simulink model "ex_longlat_dynamics_with_tire"  (R2026a)
settings: Solver=VariableStepAuto
libraries: aerolibconvert2 x2
settings Model: Creator=doyeop  LastModifiedBy=doyeop

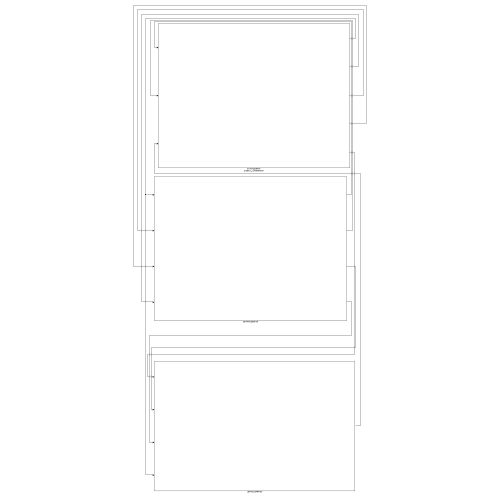
[thumbnail: Simulink's stored preview of the top-level diagram]
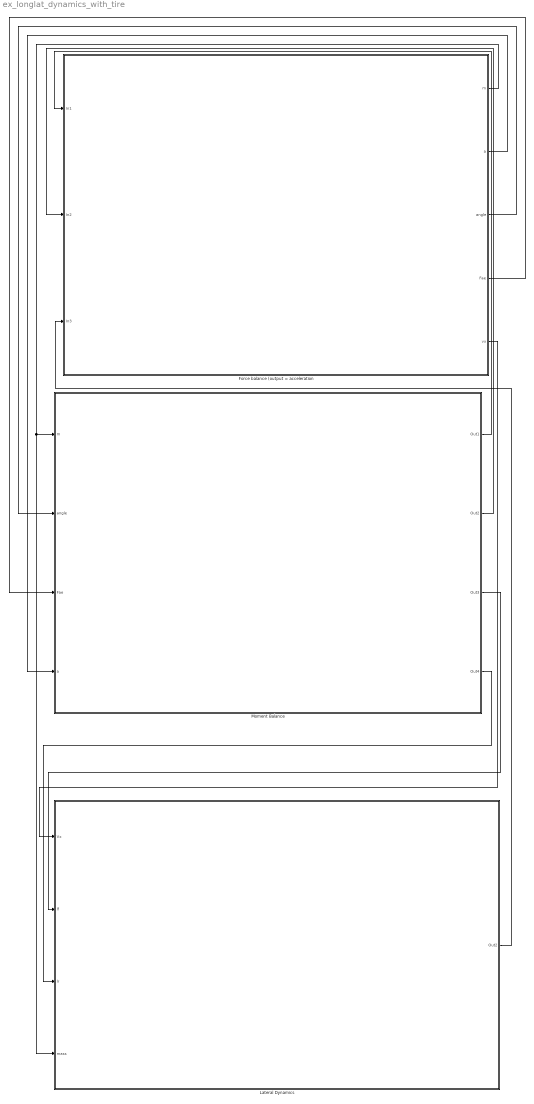
== system ex_longlat_dynamics_with_tire ==
  Force balance (output = acceleration : Subsystem
  Lateral Dynamics : Subsystem
  Moment Balance : Subsystem
  wires:
  Force balance (output = acceleration/1(m) -> Lateral Dynamics/4(mass), Moment Balance/1(m)
  Force balance (output = acceleration/2(a) -> Moment Balance/4(a)
  Force balance (output = acceleration/3(angle) -> Moment Balance/2(angle)
  Force balance (output = acceleration/4(Fae) -> Moment Balance/3(Fae)
  Moment Balance/1(Out1) -> Force balance (output = acceleration/1(In1)
  Moment Balance/2(Out2) -> Force balance (output = acceleration/2(In2)
  Force balance (output = acceleration/5(vx) -> Lateral Dynamics/1(Vx)
  Moment Balance/3(Out3) -> Lateral Dynamics/2(lf)
  Moment Balance/4(Out4) -> Lateral Dynamics/3(lr)
  Lateral Dynamics/1(Out2) -> Force balance (output = acceleration/3(In3)

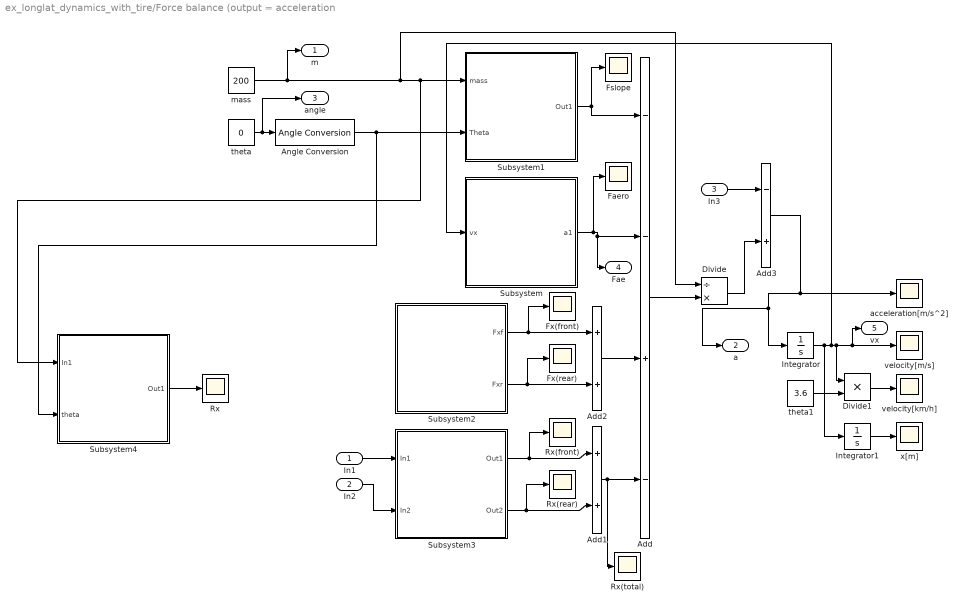
== system ex_longlat_dynamics_with_tire/Force balance (output = acceleration ==
  In1 : Inport
  In2 : Inport  Port=2
  In3 : Inport  Port=3
  Add : Sum  Inputs=--+-
  Add1 : Sum
  Add2 : Sum
  Add3 : Sum  Inputs=-+
  Angle Conversion : aerolibconvert2/Angle Conversion  IU=deg  OU=rad
  Divide : Product  Inputs=/*
  Divide1 : Product  Inputs=**
  Faero : Scope
      settings: ActiveDisplayYMinimum=-21.806973838724872  ActiveDisplayYMaximum=245.93181269445461  DataLoggingVariableName=ScopeData4
  Fslope : Scope
      settings: ActiveDisplayYMinimum=467.68768501992645  ActiveDisplayYMaximum=4126.826484026702  DataLoggingVariableName=ScopeData3
  Fx(front) : Scope
      settings: ActiveDisplayYMinimum=-0.77322383064043154  ActiveDisplayYMaximum=0.91988628090500946  DataLoggingVariableName=ScopeData5
  Fx(rear) : Scope
      settings: ActiveDisplayYMinimum=-0.77322383064043154  ActiveDisplayYMaximum=0.91988628090500946  DataLoggingVariableName=ScopeData10
  Integrator : Integrator
  Integrator1 : Integrator
  Rx : Scope
      settings: ActiveDisplayYMinimum=21.392000000000003  ActiveDisplayYMaximum=41.392  DataLoggingVariableName=ScopeData6
  Rx(front) : Scope
      settings: ActiveDisplayYMinimum=-1  ActiveDisplayYMaximum=1  DataLoggingVariableName=ScopeData11
  Rx(rear) : Scope
      settings: ActiveDisplayYMinimum=-1  ActiveDisplayYMaximum=1  DataLoggingVariableName=ScopeData12
  Rx(total) : Scope
      settings: ActiveDisplayYMinimum=26.459225679325527  ActiveDisplayYMaximum=38.083177364358953  DataLoggingVariableName=ScopeData13
  Subsystem : Subsystem
  Subsystem1 : Subsystem
  Subsystem2 : Subsystem
  Subsystem3 : Subsystem
  Subsystem4 : Subsystem
  acceleration[m/s^2] : Scope
      settings: ActiveDisplayYMinimum=-1  ActiveDisplayYMaximum=1
  mass : Constant  Value=200  SampleTime=-1
  theta : Constant  Value=0  SampleTime=-1
  theta1 : Constant  Value=3.6  SampleTime=-1
  velocity[km/h] : Scope
      settings: ActiveDisplayYMinimum=-12.890564976943338  ActiveDisplayYMaximum=101.85529757372632  DataLoggingVariableName=ScopeData7
  velocity[m/s] : Scope
      settings: ActiveDisplayYMinimum=-1  ActiveDisplayYMaximum=1
  x[m] : Scope
      settings: ActiveDisplayYMinimum=-1  ActiveDisplayYMaximum=1  DataLoggingVariableName=ScopeData2
  m : Outport
  a : Outport  Port=2
  angle : Outport  Port=3
  Fae : Outport  Port=4
  vx : Outport  Port=5
  wires:
  Divide1/1 -> velocity[km/h]/1
  Subsystem/1(a1) -> Faero/1, Add/2, Fae/1
  Integrator1/1 -> x[m]/1
  Add/1 -> Divide/2
  Angle Conversion/1 -> Subsystem4/2(theta), Subsystem1/2(Theta)
  mass/1 -> m/1, Divide/1, Subsystem4/1(In1), Subsystem1/1(mass)
  Subsystem2/1(Fxf) -> Add2/1, Fx(front)/1
  theta1/1 -> Divide1/2
  Integrator/1 -> Integrator1/1, Subsystem/1(vx), Divide1/1, vx/1, velocity[m/s]/1
  Subsystem1/1(Out1) -> Fslope/1, Add/1
  Subsystem4/1(Out1) -> Rx/1
  theta/1 -> angle/1, Angle Conversion/1
  Subsystem2/2(Fxr) -> Fx(rear)/1, Add2/2
  In1/1 -> Subsystem3/1(In1)
  In2/1 -> Subsystem3/2(In2)
  Add1/1 -> Add/4, Rx(total)/1
  Subsystem3/2(Out2) -> Rx(rear)/1, Add1/2
  Subsystem3/1(Out1) -> Rx(front)/1, Add1/1
  Add2/1 -> Add/3
  In3/1 -> Add3/1
  Divide/1 -> Add3/2
  Add3/1 -> acceleration[m/s^2]/1, a/1, Integrator/1

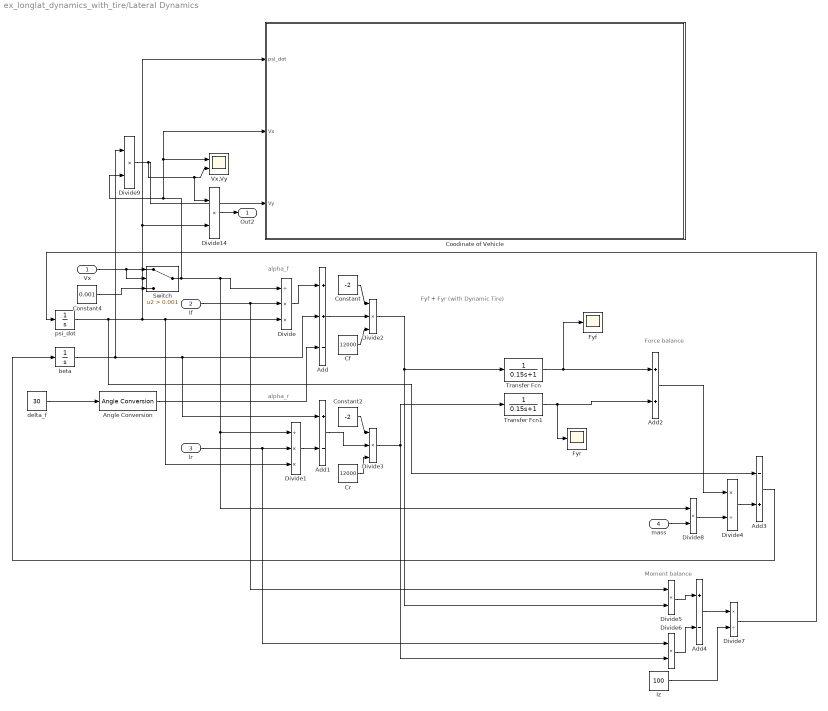
== system ex_longlat_dynamics_with_tire/Lateral Dynamics ==
  note: Moment balance
  note: Force balance
  note: Fyf + Fyr (with Dynamic Tire)
  note: alpha_r
  note: alpha_f
  Vx : Inport
  lf : Inport  Port=2
  lr : Inport  Port=3
  mass : Inport  Port=4
  Add : Sum  Inputs=++-
  Add1 : Sum  Inputs=+-
  Add2 : Sum
  Add3 : Sum  Inputs=-+
  Add4 : Sum  Inputs=+-
  Angle Conversion : aerolibconvert2/Angle Conversion  IU=deg  OU=rad
  Cf : Constant  Value=12000  SampleTime=-1
  Constant : Constant  Value=-2  SampleTime=-1
  Constant2 : Constant  Value=-2  SampleTime=-1
  Constant4 : Constant  Value=0.001
  Coodinate of Vehicle : Subsystem
  Cr : Constant  Value=12000  SampleTime=-1
  Divide : Product  Inputs=/**
  Divide1 : Product  Inputs=/**
  Divide{5..6,8..9,14} (5 alike) : Product  Inputs=**
  Divide2 : Product  Inputs=***
  Divide3 : Product  Inputs=***
  Divide4 : Product  Inputs=*/
  Divide7 : Product  Inputs=*/
  Fyf : Scope
      settings: ActiveDisplayYMinimum=-1407.4048741262529  ActiveDisplayYMaximum=11639.532558539519  DataLoggingVariableName=ScopeData14
  Fyr : Scope
      settings: ActiveDisplayYMinimum=-970.12534509010345  ActiveDisplayYMaximum=7745.6964021526865  DataLoggingVariableName=ScopeData15
  Iz : Constant  Value=100  SampleTime=-1
  Switch : Switch  Criteria=u2 > Threshold  Threshold=0.001  SaturateOnIntegerOverflow=off  InputSameDT=off
  Transfer Fcn : TransferFcn  Denominator=[0.15 1]
  Transfer Fcn1 : TransferFcn  Denominator=[0.15 1]
  Vx,Vy : Scope  NumInputPorts=2
      settings: ActiveDisplayYMinimum=-0.62237224027035509  ActiveDisplayYMaximum=5.6013501624331967  DataLoggingVariableName=ScopeData16
  beta : Integrator
  delta_f : Constant  Value=30
  psi_dot : Integrator
  Out2 : Outport
  wires:
  beta/1 -> Add/2, Add1/1, Divide9/1
  Divide/1 -> Add/1
  Angle Conversion/1 -> Add/3
  lr/1 -> Divide6/1, Divide1/2
  Divide1/1 -> Add1/2
  Constant/1 -> Divide2/1
  Add/1 -> Divide2/2
  Cf/1 -> Divide2/3
  Add1/1 -> Divide3/2
  Constant2/1 -> Divide3/1
  Cr/1 -> Divide3/3
  Divide2/1 -> Transfer Fcn/1, Divide5/2
  Divide3/1 -> Divide6/2, Transfer Fcn1/1
  Divide4/1 -> Add3/2
  Add3/1 -> beta/1
  lf/1 -> Divide5/1, Divide/2
  Divide5/1 -> Add4/1
  Divide6/1 -> Add4/2
  Add4/1 -> Divide7/1
  Iz/1 -> Divide7/2
  Divide7/1 -> psi_dot/1
  Vx/1 -> Switch/2, Switch/1
  Constant4/1 -> Switch/3
  mass/1 -> Divide8/2
  Divide8/1 -> Divide4/2
  Add2/1 -> Divide4/1
  delta_f/1 -> Angle Conversion/1
  Transfer Fcn/1 -> Fyf/1, Add2/1
  Transfer Fcn1/1 -> Fyr/1, Add2/2
  Switch/1 -> Divide8/1, Divide1/1, Divide/1, Divide9/2, Coodinate of Vehicle/2(Vx), Vx,Vy/1
  Divide9/1 -> Divide14/1, Vx,Vy/2, Coodinate of Vehicle/3(Vy)
  psi_dot/1 -> Add3/1, Divide14/2, Coodinate of Vehicle/1(psi_dot), Divide1/3, Divide/3
  Divide14/1 -> Out2/1

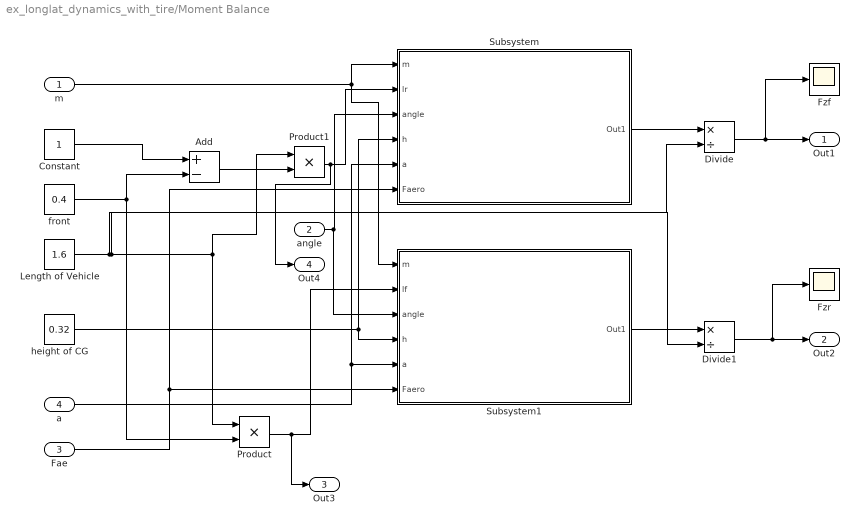
== system ex_longlat_dynamics_with_tire/Moment Balance ==
  m : Inport
  angle : Inport  Port=2
  Fae : Inport  Port=3
  a : Inport  Port=4
  Add : Sum  Inputs=+-
  Constant : Constant
  Divide : Product  Inputs=*/
  Divide1 : Product  Inputs=*/
  Fzf : Scope
      settings: ActiveDisplayYMinimum=684.79999999999961  ActiveDisplayYMaximum=684.80000000000007  DataLoggingVariableName=ScopeData8
  Fzr : Scope
      settings: DataLoggingVariableName=ScopeData9
  Length of Vehicle : Constant  Value=1.6  SampleTime=-1
  Product : Product
  Product1 : Product
  Subsystem : Subsystem
  Subsystem1 : Subsystem
  front : Constant  Value=0.4  SampleTime=-1
  height of CG : Constant  Value=0.32
  Out1 : Outport
  Out2 : Outport  Port=2
  Out3 : Outport  Port=3
  Out4 : Outport  Port=4
  wires:
  m/1 -> Subsystem1/1(m), Subsystem/1(m)
  angle/1 -> Subsystem1/3(angle), Subsystem/3(angle)
  front/1 -> Product/2, Add/2
  Constant/1 -> Add/1
  Length of Vehicle/1 -> Divide/2, Divide1/2, Product1/1, Product/1
  Add/1 -> Product1/2
  Product1/1 -> Out4/1, Subsystem/2(lr)
  height of CG/1 -> Subsystem/4(h), Subsystem1/4(h)
  a/1 -> Subsystem1/5(a), Subsystem/5(a)
  Fae/1 -> Subsystem1/6(Faero), Subsystem/6(Faero)
  Subsystem/1(Out1) -> Divide/1
  Subsystem1/1(Out1) -> Divide1/1
  Product/1 -> Out3/1, Subsystem1/2(lf)
  Divide/1 -> Out1/1, Fzf/1
  Divide1/1 -> Fzr/1, Out2/1

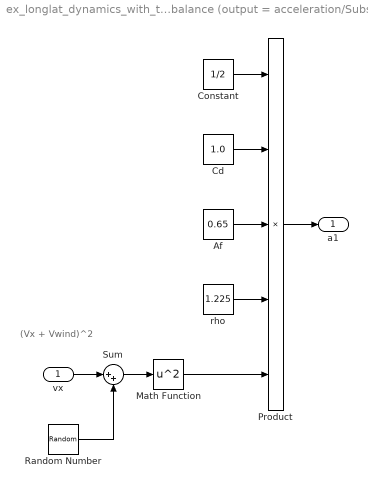
== system ex_longlat_dynamics_with_tire/Force balance (output = acceleration/Subsystem ==
  note: (Vx + Vwind)^2
  vx : Inport
  Af : Constant  Value=0.65  SampleTime=-1
  Cd : Constant  Value=1.0  SampleTime=-1
  Constant : Constant  Value=1/2  SampleTime=-1
  Math Function : Math  Operator=square
  Product : Product  Inputs=5
  Random Number : RandomNumber  Mean=3  Variance=0.5^2  SampleTime=0.1
  Sum : Sum  Inputs=|++
  rho : Constant  Value=1.225  SampleTime=-1
  a1 : Outport
  wires:
  Cd/1 -> Product/2
  Af/1 -> Product/3
  Constant/1 -> Product/1
  rho/1 -> Product/4
  Random Number/1 -> Sum/2
  vx/1 -> Sum/1
  Sum/1 -> Math Function/1
  Math Function/1 -> Product/5
  Product/1 -> a1/1

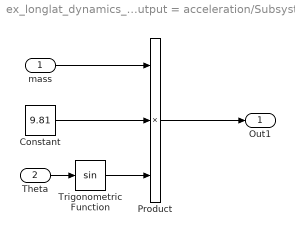
== system ex_longlat_dynamics_with_tire/Force balance (output = acceleration/Subsystem1 ==
  mass : Inport
  Theta : Inport  Port=2
  Constant : Constant  Value=9.81  SampleTime=-1
  Product : Product  Inputs=3
  Trigonometric Function : Trigonometry
  Out1 : Outport
  wires:
  mass/1 -> Product/1
  Theta/1 -> Trigonometric Function/1
  Trigonometric Function/1 -> Product/3
  Constant/1 -> Product/2
  Product/1 -> Out1/1

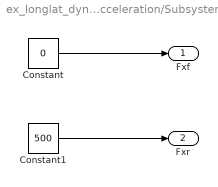
== system ex_longlat_dynamics_with_tire/Force balance (output = acceleration/Subsystem2 ==
  Constant : Constant  Value=0  SampleTime=-1
  Constant1 : Constant  Value=500  SampleTime=-1
  Fxf : Outport
  Fxr : Outport  Port=2
  wires:
  Constant/1 -> Fxf/1
  Constant1/1 -> Fxr/1

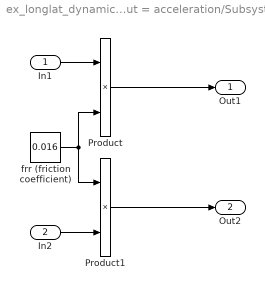
== system ex_longlat_dynamics_with_tire/Force balance (output = acceleration/Subsystem3 ==
  In1 : Inport
  In2 : Inport  Port=2
  Product : Product
  Product1 : Product
  frr (friction coefficient) : Constant  Value=0.016  SampleTime=-1
  Out1 : Outport
  Out2 : Outport  Port=2
  wires:
  In1/1 -> Product/1
  frr (friction coefficient)/1 -> Product/2, Product1/1
  In2/1 -> Product1/2
  Product/1 -> Out1/1
  Product1/1 -> Out2/1

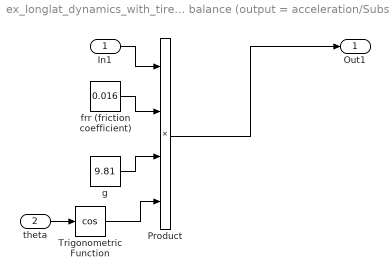
== system ex_longlat_dynamics_with_tire/Force balance (output = acceleration/Subsystem4 ==
  In1 : Inport
  theta : Inport  Port=2
  Product : Product  Inputs=4
  Trigonometric Function : Trigonometry  Operator=cos
  frr (friction coefficient) : Constant  Value=0.016  SampleTime=-1
  g : Constant  Value=9.81  SampleTime=-1
  Out1 : Outport
  wires:
  In1/1 -> Product/1
  frr (friction coefficient)/1 -> Product/2
  g/1 -> Product/3
  theta/1 -> Trigonometric Function/1
  Product/1 -> Out1/1
  Trigonometric Function/1 -> Product/4

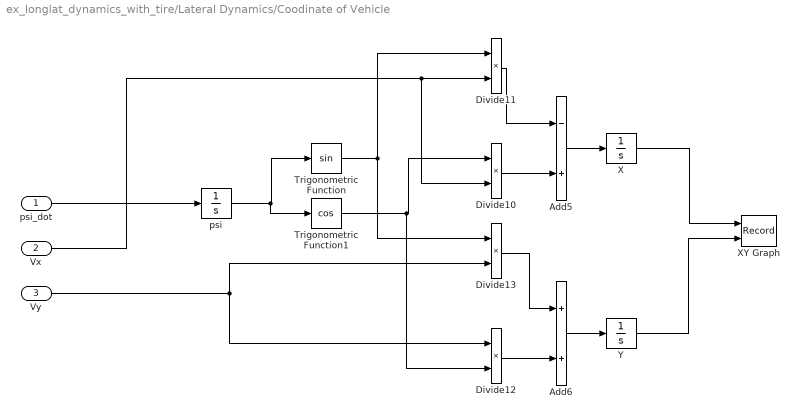
== system ex_longlat_dynamics_with_tire/Lateral Dynamics/Coodinate of Vehicle ==
  psi_dot : Inport
  Vx : Inport  Port=2
  Vy : Inport  Port=3
  Add5 : Sum  Inputs=-+
  Add6 : Sum
  Divide{10..13} (4 alike) : Product  Inputs=**
  Trigonometric Function : Trigonometry
  Trigonometric Function1 : Trigonometry  Operator=cos
  X : Integrator
  XY Graph : Record  NumPorts=2.0  FileSettingsInternal="{\"entries\":[{\"content\":{\"excelSettings\":{\"content\":{},\"type\":\"Streamout.ExcelSettings\"},\"parquetSettings\":{\"content\":{},\"type\":\"Streamout.ParquetSettings\"}},\"type\":\"Streamout.FileSettingStorage\",\"uuid\":\"\"}],\"packageUris\":[\"http:\\/\\/schema.mathworks.com\\/mf0\\/streamout_blocks\\/R2020a\"],\"version\":\"1.0\"}"  FrameSettings=[0, 0]  Layout=[1 1]  SignalsInternal="{\"entries\":[{\"content\":{\"signals\":[{\"content\":{\"blockPath\":[],\"dimensions\":[1],\"domain\":\"\",\"lineColor\":\"#a2142f\",\"plots\":[ 1 ],\"port\":1,\"signalID\":1,\"signalName\":\"X\"},\"type\":\"RecordBlkView.Signal\",\"uuid\":\"\"},{\"content\":{\"blockPath\":[],\"dimensions\":[1],\"domain\":\"\",\"lineColor\":\"#139fff\",\"plots\":[ 1 ],\"port\":2,\"signalID\":2,\"signalName\":\"Y\"},\"type\":\"RecordBlkView.Signal\",\"uuid\":\"\"}]},\"type\":\"RecordBlkView.InputSignals\",\"uuid\":\"\"}],\"packageUris\":[\"http:\\/\\/schema.mathworks.com\\/mf0\\/streamout_blocks\\/R2020a\"],\"version\":\"1.0\"}"  VisualizationBindings="{\"xyplotplugin\":{\"info\":[{\"series\":[{\"bindingParametersList\":[{\"parameter\":\"X-Axis\",\"signalID\":1,\"signalName\":\"X\"},{\"parameter\":\"Y-Axis\",\"signalID\":2,\"signalName\":\"Y\"}],\"seriesID\":0}],\"subplotID\":1}]}}"  CompatibilityTag=XY
  Y : Integrator
  psi : Integrator
  wires:
  X/1 -> XY Graph/1
  Add6/1 -> Y/1
  Divide10/1 -> Add5/2
  psi/1 -> Trigonometric Function1/1, Trigonometric Function/1
  Divide12/1 -> Add6/2
  Trigonometric Function1/1 -> Divide12/2, Divide10/1
  Y/1 -> XY Graph/2
  Divide13/1 -> Add6/1
  psi_dot/1 -> psi/1
  Add5/1 -> X/1
  Trigonometric Function/1 -> Divide11/1, Divide13/1
  Divide11/1 -> Add5/1
  Vx/1 -> Divide10/2, Divide11/2
  Vy/1 -> Divide12/1, Divide13/2

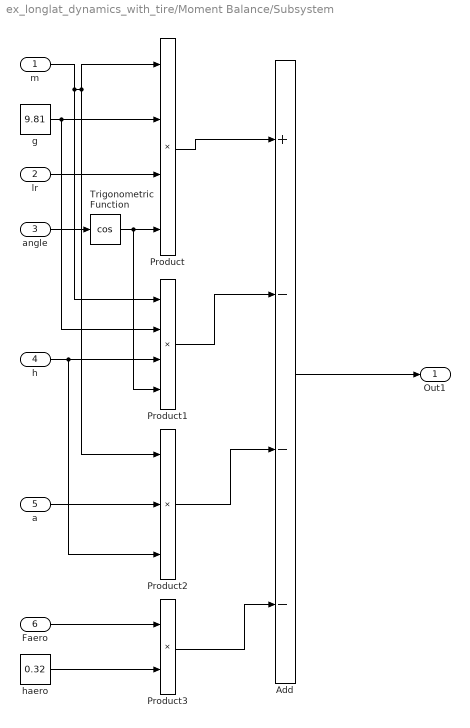
== system ex_longlat_dynamics_with_tire/Moment Balance/Subsystem ==
  m : Inport
  lr : Inport  Port=2
  angle : Inport  Port=3
  h : Inport  Port=4
  a : Inport  Port=5
  Faero : Inport  Port=6
  Add : Sum  Inputs=+---
  Product : Product  Inputs=4
  Product1 : Product  Inputs=4
  Product2 : Product  Inputs=3
  Product3 : Product
  Trigonometric Function : Trigonometry  Operator=cos
  g : Constant  Value=9.81  SampleTime=-1
  haero : Constant  Value=0.32  SampleTime=-1
  Out1 : Outport
  wires:
  m/1 -> Product1/1, Product2/1, Product/1
  angle/1 -> Trigonometric Function/1
  g/1 -> Product1/2, Product/2
  lr/1 -> Product/3
  Trigonometric Function/1 -> Product1/4, Product/4
  a/1 -> Product2/2
  h/1 -> Product2/3, Product1/3
  haero/1 -> Product3/2
  Faero/1 -> Product3/1
  Product/1 -> Add/1
  Product1/1 -> Add/2
  Product2/1 -> Add/3
  Product3/1 -> Add/4
  Add/1 -> Out1/1

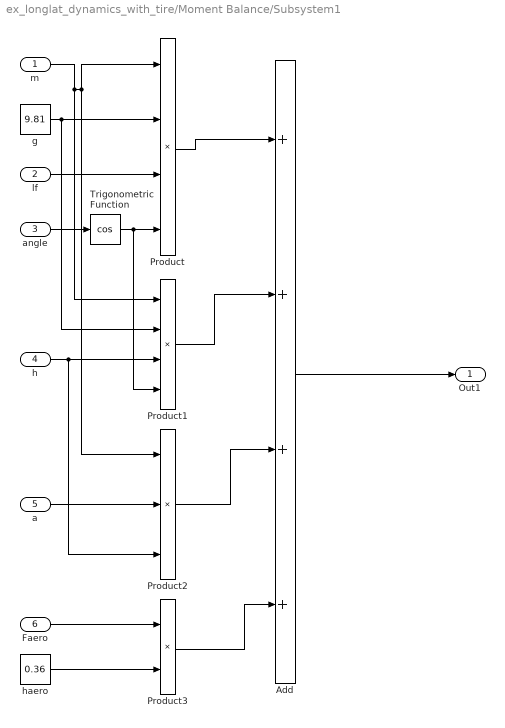
== system ex_longlat_dynamics_with_tire/Moment Balance/Subsystem1 ==
  m : Inport
  lf : Inport  Port=2
  angle : Inport  Port=3
  h : Inport  Port=4
  a : Inport  Port=5
  Faero : Inport  Port=6
  Add : Sum  Inputs=++++
  Product : Product  Inputs=4
  Product1 : Product  Inputs=4
  Product2 : Product  Inputs=3
  Product3 : Product
  Trigonometric Function : Trigonometry  Operator=cos
  g : Constant  Value=9.81  SampleTime=-1
  haero : Constant  Value=0.36  SampleTime=-1
  Out1 : Outport
  wires:
  m/1 -> Product1/1, Product2/1, Product/1
  angle/1 -> Trigonometric Function/1
  g/1 -> Product1/2, Product/2
  lf/1 -> Product/3
  Trigonometric Function/1 -> Product1/4, Product/4
  a/1 -> Product2/2
  h/1 -> Product2/3, Product1/3
  haero/1 -> Product3/2
  Faero/1 -> Product3/1
  Product/1 -> Add/1
  Product1/1 -> Add/2
  Product2/1 -> Add/3
  Product3/1 -> Add/4
  Add/1 -> Out1/1
